simulink model "level_tank"  (R2023b)
settings: Solver=VariableStepAuto  StartTime=0.0  StopTime=350  RelTol=1e-3
undefined symbols (not defined in the file): daq
libraries: daqlib x2, simulink x1, fuzblock x1, dspstat3 x1
settings Model: Creator=ccm-stu  LastModifiedBy=HP

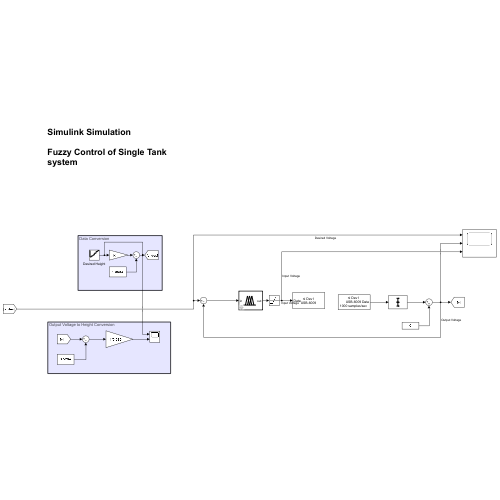
[thumbnail: Simulink's stored preview of the top-level diagram]
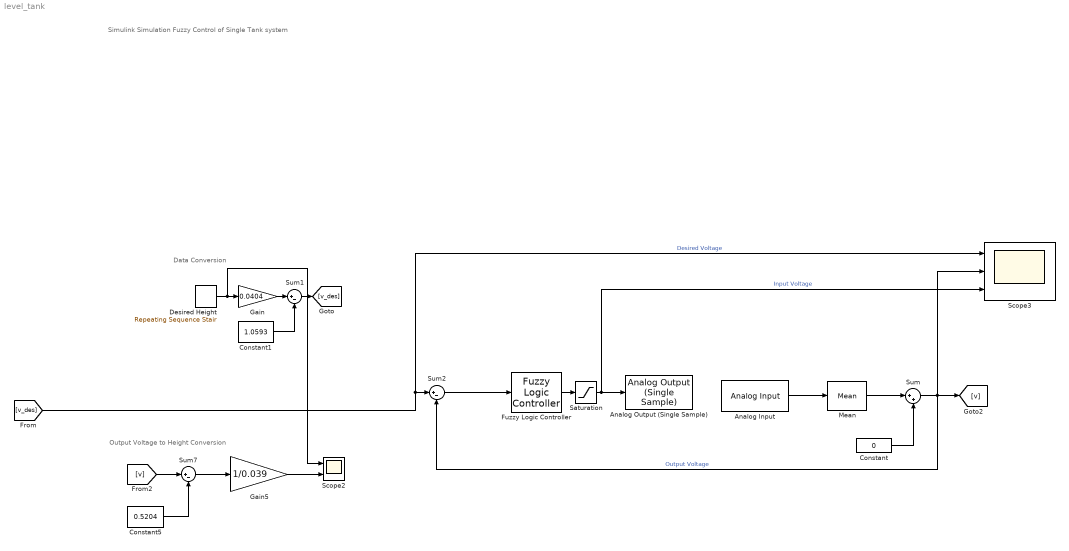
== system level_tank ==
  note: Simulink Simulation
      |
      | Fuzzy Control of Single Tank system
  note: Output Voltage to Height Conversion
  note: Data Conversion
  Analog Input : daqlib/Analog Input  DeviceMenu=(none)  Device=ni Dev1 (USB-6009)  ObjConstructor=daq.createSession('ni')  NChannelsSelected=1  Channels=1$ai0$$Dev1$1$8$2$1$#0$ai1$$Dev1$1$8$2$1$#0$ai2$$Dev1$1$8$2$1$#0$ai3$$Dev1$1$8$2$1$#0$ai4$$Dev1$1$7$1$1$#0$ai5$$Dev1$1$7$1$1$#0$ai6$$Dev1$1$7$1$1$#0$ai7$$Dev1$1$7$1$1$#  NPorts=1 for all channels  SampleRate=1000  ActualRate=1000  ScansPerTrigger=50  OutputTimestamp=off  AcqMode=0  NumFrameBuffer=100  OutputTriggertime=off
  Analog Output (Single Sample) : daqlib/Analog Output (Single Sample)  DeviceMenu=(none)  Device=ni Dev1 (USB-6009)  ObjConstructor=daq.createSession('ni')  NChannelsSelected=1  Channels=0$ao0$$Dev1$1$1$N/A$#1$ao1$$Dev1$1$1$N/A$#  NPorts=1 for all channels  BlockSampleTime=1
  Constant : Constant  Value=0
  Constant1 : Constant  Value=1.0593
  Constant5 : Constant  Value=0.5204
  Desired Height : simulink/Sources/Repeating Sequence Stair  OutValues=[50 70 90 120 150 170].'  tsamp=70  OutMin=[]  OutMax=[]  OutDataTypeStr=double  OutputDataTypeScalingMode=double  OutDataType=fixdt(0,8)  ConRadixGroup=Best Precision: Vector-wise  OutScaling=2^-12
  Fuzzy Logic Controller : fuzblock/Fuzzy Logic  Controller  FIS='fiscoupledtank_1.fis'  OutputSampleNumber=101  DataType=double  FuzzifiedInputs=off  RuleFiringStrengths=off  RuleOutputs=off  AggregatedOutputs=off  SimulateUsing=Interpreted execution  OutOfRangeInputValueMessage=warning  NoRuleFiredMessage=warning  EmptyOutputFuzzySetMessage=warning
  Gain : Gain  Gain=0.0404
  Gain5 : Gain  Gain=1/0.039
  Mean : dspstat3/Mean  run=off  InputProcessing=Columns as channels (frame based)  reset_popup=None  directionMode=Each column  dimension=1  roiEnable=off  roiType=Rectangles  roiPortion=Entire ROI  roiOutput=Individual statistics for each ROI  roiFlag=off  roundingMode=Floor  overflowMode=off  outputDataTypeStr=Inherit: Same as accumulator  outputMin=[]  outputMax=[]  outputLastDataTypeStr=Inherit: Same as accumulator
  Saturation : Saturate  UpperLimit=5  LowerLimit=0
  Scope2 : Scope  NumInputPorts=2
  Scope3 : Scope  NumInputPorts=3
  Sum : Sum  Inputs=|++
  Sum1 : Sum  Inputs=|+-
  Sum2 : Sum  Inputs=|+-
  Sum7 : Sum  Inputs=|+-
  wires:
  Analog Input/1 -> Mean/1
  Mean/1 -> Sum/1
  Sum/1 -> [v], Scope3/2, Sum2/2  "Output Voltage"
  Constant/1 -> Sum/2
  Desired Height/1 -> Scope2/1, Gain/1
  Gain/1 -> Sum1/1
  Constant1/1 -> Sum1/2
  Sum1/1 -> [v_des]
  [v_des] -> Sum2/1, Scope3/1  "Desired Voltage"
  Saturation/1 -> Analog Output (Single Sample)/1, Scope3/3  "Input Voltage"
  [v] -> Sum7/1
  Sum7/1 -> Gain5/1
  Constant5/1 -> Sum7/2
  Gain5/1 -> Scope2/2
  Fuzzy Logic Controller/1 -> Saturation/1
  Sum2/1 -> Fuzzy Logic Controller/1
